simulink model "quat_mult"  (R2018a)
settings: Solver=VariableStepAuto  StartTime=0.0  StopTime=10.0  RelTol=1e-3
settings Model: Creator=lamy  LastModifiedBy=lamy

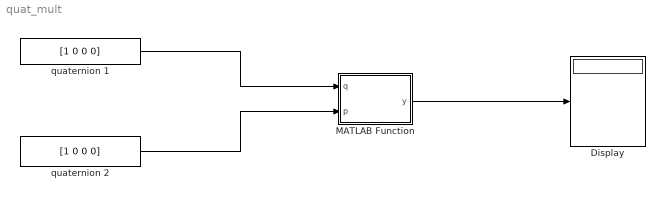
== system quat_mult ==
  Display : Display
  MATLAB Function : MATLAB Function  TreatAsAtomicUnit=on
  quaternion 1 : Constant  Value=[1 0 0 0]
  quaternion 2 : Constant  Value=[1 0 0 0]
  wires:
  MATLAB Function/1(y) -> Display/1
  quaternion 1/1 -> MATLAB Function/1(q)
  quaternion 2/1 -> MATLAB Function/2(p)

== matlab function quat_mult/MATLAB Function ==
  data: q input; y output; p input
function y = quat_mult(q, p)
qo=q(1);
qvec=q(2:4);
po=p(1);
pvec=p(2:4);
yo = qo*po - dot(qvec,pvec);
yvec = po*qvec + qo*pvec + cross(pvec,qvec);
y = [yo; yvec];
